simulink model "modelBCPWM"  (R2024a)
settings: Solver=ode23tb  StartTime=0.0  StopTime=0.05  MaxStep=sover_max_step  RelTol=1e-5
values from neighbouring files (symbols this model uses):
  BLDC_120_180 = 1    [initBCPWM.m]
  duty_cycle = 0.6    [initBCPWM.m]
  f_fundamental = 265    [initBCPWM.m]    (also in initSVPWM.m = 100)
  f_pwm = 20000    [initBCPWM.m]    (also in initSVPWM.m)
  Ke = sqrt(2) * 3.35e-3 * 60 / 2 / pi / p    [initBCPWM.m]    (also in initSVPWM.m)
  load_angle = pi/6    (= 0.523598775598)    [initBCPWM.m]    (also in initSVPWM.m = load_angle_offset - voltage_angle)
  Ls = 3/2 * 1.2e-3    (= 0.0018)    [initBCPWM.m]    (also in initSVPWM.m)
  Rs = 3/2 * 0.8    (= 1.2)    [initBCPWM.m]    (also in initSVPWM.m)
  sover_max_step = 1e-6    (= 1e-06)    [initBCPWM.m]    (also in initSVPWM.m)
  Vdc = 24    [initBCPWM.m]    (also in initSVPWM.m)
libraries: simulink x16, spsSeriesRLCBranchLib x6, spsMosfetLib x6, spsVoltageMeasurementLib x5, spsNeutralLib x4, spsControlledVoltageSourceLib x3, spsGroundLib x3, spsCurrentMeasurementLib x1, spsDCVoltageSourceLib x1, sps_lib x1
settings Model: SimulationMode=accelerator  Creator=mandr  LastModifiedBy=danielmcguiness
settings SolverCC: ZeroCrossControl=EnableAll  AlgebraicLoopSolver=TrustRegion  SolverResetMethod=Robust
settings DebuggingCC: UnconnectedInputMsg=warning  UnconnectedOutputMsg=warning  UnconnectedLineMsg=warning
settings ModelReferenceCC: EnableRefExpFcnMdlSchedulingChecks=on
settings RTWCC: GPUComputeCapability=3.5

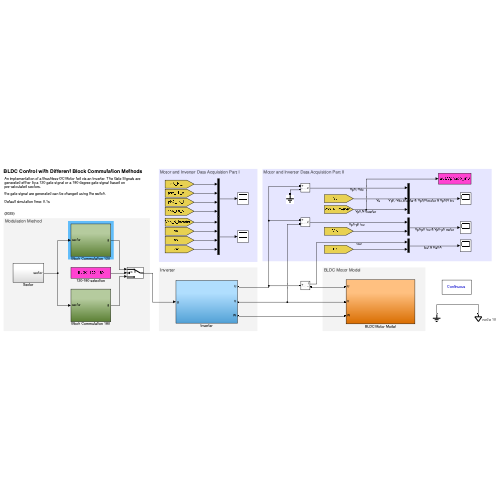
[thumbnail: Simulink's stored preview of the top-level diagram]
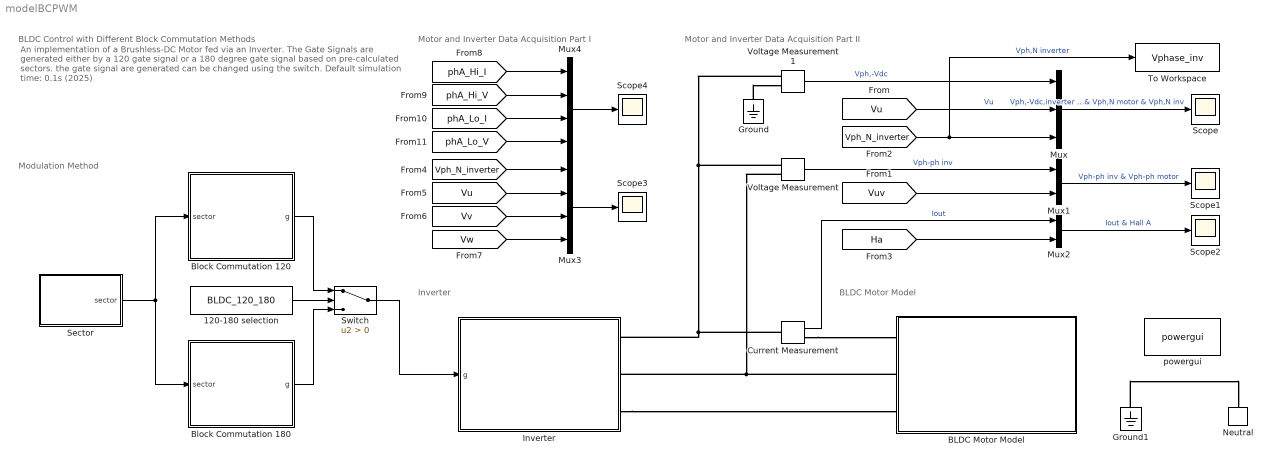
== system modelBCPWM ==
  note: An implementation of a Brushless-DC Motor fed via an Inverter. The Gate Signals are generated either by a 120 gate signal or a 180 degree gate signal based on
      | pre-calculated sectors.
      | the gate signal are generated can be changed using the switch.
      | Default simulation time: 0.1s
      |
      | (2025)
  note: BLDC Control with Different Block Commutation Methods
  note: BLDC Motor Model
  note: Motor and Inverter Data Acquisition Part II
  note: Motor and Inverter Data Acquisition Part I
  note: Inverter
  note: Modulation Method
  120-180 selection : Constant  Value=BLDC_120_180
  BLDC Motor Model : Subsystem
  Block Commutation 120 : Subsystem
  Block Commutation 180 : Subsystem
  Current Measurement : spsCurrentMeasurementLib/Current Measurement  PhasorSimulation=off  OutputType=Complex  PSBequivalent=0
  Ground : spsGroundLib/Ground  LConnTagsString=a
  Ground1 : spsGroundLib/Ground  LConnTagsString=a
  Inverter : Subsystem
  Mux : Mux  Inputs=3
  Mux1 : Mux  Inputs=2
  Mux2 : Mux  Inputs=2
  Mux3 : Mux
  Mux4 : Mux
  Neutral : spsNeutralLib/Neutral  LConnTagsString=a  NodeNumber=10
      settings: AttributesFormatString=node %<NodeNumber>  LibrarySourceBlock=sps_lib/Utilities/Neutral
  Scope{,1..4} (5 alike) : Scope
  Sector : Subsystem
  Switch : Switch  Criteria=u2 > Threshold  SaturateOnIntegerOverflow=off  InputSameDT=off
  To Workspace : ToWorkspace  VariableName=Vphase_inv  SaveFormat=Timeseries  SampleTime=sover_max_step
  Voltage Measurement : spsVoltageMeasurementLib/Voltage Measurement  PhasorSimulation=off  OutputType=Complex  PSBequivalent=0
  Voltage Measurement1 : spsVoltageMeasurementLib/Voltage Measurement  PhasorSimulation=off  OutputType=Complex  PSBequivalent=0
  powergui : sps_lib/powergui  Priority=1  SimulationMode=Continuous  SampleTime=50e-6  frequency=60  Iterations=50  frequencyindice=0  Pbase=100e6  ErrMax=1e-4  UnitsV=kV  UnitsW=MW  buscounter=0  FunctionMessages=off  echomessages=off  EnableUseOfTLC=off  CurrentSourceSwitches=off  DisableSnubberDevices=off  DisableRonSwitches=off  DisableVfSwitches=off  DisplayEquations=off  AutomaticDiscreteSolvers=off  SolverType=Tustin/Backward Euler (TBE)  Interpol=off  ExternalGateDelay=off  methode=off  Ts=100  x0status=blocks  SPID=on  SwTol=0  HookPort=off  NonlinearTolerance=1e-4  nMaxIteration=100  ContinueOnMaxIteration=off  RestoreLinks=warning  ResistiveCurrentMeasurement=off  Frange=[0:2:500]  Ylog=off  Xlog=on  ShowGrid=off  save=off  variable=ZData  structure=0  ZoomFFT=off  StartTime=0.0  cycles=1  DisplayStyle=1  fundamental=60  FreqAxis=off  MaxFrequency=1000  frequencyindicesteady=1  RmsSteady=1  display=off
  wires:
  Voltage Measurement1/1 -> Mux/1  "Vph,-Vdc"
  Voltage Measurement/1 -> Mux1/1  "Vph-ph inv"
  Current Measurement/1 -> Mux2/1  "Iout"
  Mux/1 -> Scope/1  "Vph,-Vdc,inverter & Vph,N motor & Vph,N inv"
  [Vu] -> Mux/2  "Vu"
  Mux1/1 -> Scope1/1  "Vph-ph inv & Vph-ph motor"
  [Vuv] -> Mux1/2
  [Vph_N_inverter] -> To Workspace/1, Mux/3  "Vph,N inverter"
  Mux2/1 -> Scope2/1  "Iout & Hall A"
  [Ha] -> Mux2/2
  Switch/1 -> Inverter/1(g)
  Block Commutation 180/1(g) -> Switch/3
  Block Commutation 120/1(g) -> Switch/1
  120-180 selection/1 -> Switch/2
  [Vph_N_inverter] -> Mux3/1
  Mux3/1 -> Scope3/1
  [Vu] -> Mux3/2
  [Vv] -> Mux3/3
  [Vw] -> Mux3/4
  Sector/1(sector) -> Block Commutation 180/1(sector), Block Commutation 120/1(sector)
  [phA_Hi_I] -> Mux4/1
  [phA_Hi_V] -> Mux4/2
  [phA_Lo_I] -> Mux4/3
  [phA_Lo_V] -> Mux4/4
  Mux4/1 -> Scope4/1
  connections:
  Voltage Measurement/LConn1 -- Current Measurement/LConn1 -- Inverter/RConn1 -- Voltage Measurement1/LConn1
  Voltage Measurement/LConn2 -- BLDC Motor Model/LConn2 -- Inverter/RConn2
  Ground/LConn1 -- Voltage Measurement1/LConn2
  Current Measurement/RConn1 -- BLDC Motor Model/LConn1
  Inverter/RConn3 -- BLDC Motor Model/LConn3
  Ground1/LConn1 -- Neutral/LConn1

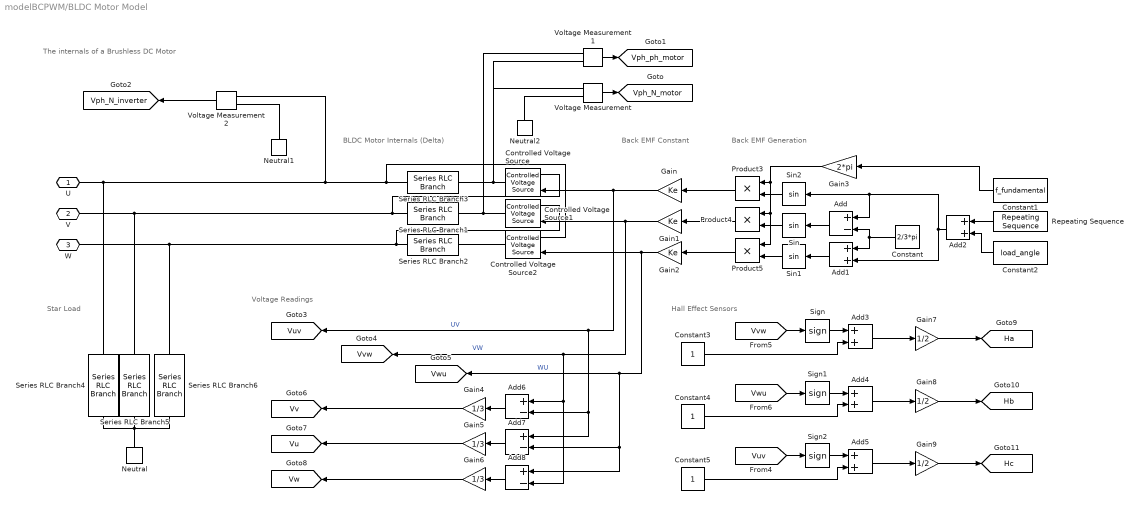
== system modelBCPWM/BLDC Motor Model ==
  note: The internals of a Brushless DC Motor
  note: Back EMF Generation
  note: Back EMF Constant
  note: Star Load
  note: Voltage Readings
  note: Hall Effect Sensors
  note: BLDC Motor Internals (Delta)
  Add{,6..8} (4 alike) : Sum  Inputs=+-
  Add{1..5} (5 alike) : Sum
  Constant : Constant  Value=2/3*pi
  Constant1 : Constant  Value=f_fundamental
  Constant2 : Constant  Value=load_angle
  Constant3 : Constant
  Constant4 : Constant
  Constant5 : Constant
  Controlled Voltage Source : spsControlledVoltageSourceLib/Controlled Voltage Source  Initialize=on  Source_Type=AC  Amplitude=0  Phase=0  Frequency=0  Measurements=None
  Controlled Voltage Source1 : spsControlledVoltageSourceLib/Controlled Voltage Source  Initialize=on  Source_Type=AC  Amplitude=0  Phase=0  Frequency=0  Measurements=None
  Controlled Voltage Source2 : spsControlledVoltageSourceLib/Controlled Voltage Source  Initialize=on  Source_Type=AC  Amplitude=0  Phase=0  Frequency=0  Measurements=None
  Gain : Gain  Gain=Ke
  Gain1 : Gain  Gain=Ke
  Gain2 : Gain  Gain=Ke
  Gain3 : Gain  Gain=2*pi
  Gain4 : Gain  Gain=1/3
  Gain5 : Gain  Gain=1/3
  Gain6 : Gain  Gain=1/3
  Gain7 : Gain  Gain=1/2
  Gain8 : Gain  Gain=1/2
  Gain9 : Gain  Gain=1/2
  Neutral : spsNeutralLib/Neutral  LConnTagsString=a  NodeNumber=10
      settings: AttributesFormatString=node %<NodeNumber>  LibrarySourceBlock=sps_lib/Utilities/Neutral
  Neutral1 : spsNeutralLib/Neutral  LConnTagsString=a  NodeNumber=10
      settings: AttributesFormatString=node %<NodeNumber>  LibrarySourceBlock=sps_lib/Utilities/Neutral
  Neutral2 : spsNeutralLib/Neutral  LConnTagsString=a  NodeNumber=10
      settings: AttributesFormatString=node %<NodeNumber>  LibrarySourceBlock=sps_lib/Utilities/Neutral
  Product3 : Product
  Product4 : Product
  Product5 : Product
  Repeating Sequence : simulink/Sources/Repeating Sequence  rep_seq_t=[0 1/f_fundamental]  rep_seq_y=[0 2*pi]
  Series RLC Branch1 : spsSeriesRLCBranchLib/Series RLC Branch  LConnTagsString=__new0  RConnTagsString=__new0  BranchType=RL  Resistance=Rs  Inductance=Ls  SetiL0=off  InitialCurrent=0  Capacitance=1e-6  Setx0=off  InitialVoltage=0  Measurements=None
  Series RLC Branch2 : spsSeriesRLCBranchLib/Series RLC Branch  LConnTagsString=__new0  RConnTagsString=__new0  BranchType=RL  Resistance=Rs  Inductance=Ls  SetiL0=off  InitialCurrent=0  Capacitance=1e-6  Setx0=off  InitialVoltage=0  Measurements=None
  Series RLC Branch3 : spsSeriesRLCBranchLib/Series RLC Branch  LConnTagsString=__new0  RConnTagsString=__new0  BranchType=RL  Resistance=Rs  Inductance=Ls  SetiL0=off  InitialCurrent=0  Capacitance=1e-6  Setx0=off  InitialVoltage=0  Measurements=None
  Series RLC Branch4 : spsSeriesRLCBranchLib/Series RLC Branch  LConnTagsString=__new0  RConnTagsString=__new0  BranchType=R  Resistance=1e3  Inductance=Ls  SetiL0=off  InitialCurrent=0  Capacitance=1e-6  Setx0=off  InitialVoltage=0  Measurements=None
  Series RLC Branch5 : spsSeriesRLCBranchLib/Series RLC Branch  LConnTagsString=__new0  RConnTagsString=__new0  BranchType=R  Resistance=1e3  Inductance=Ls  SetiL0=off  InitialCurrent=0  Capacitance=1e-6  Setx0=off  InitialVoltage=0  Measurements=None
  Series RLC Branch6 : spsSeriesRLCBranchLib/Series RLC Branch  LConnTagsString=__new0  RConnTagsString=__new0  BranchType=R  Resistance=1e3  Inductance=Ls  SetiL0=off  InitialCurrent=0  Capacitance=1e-6  Setx0=off  InitialVoltage=0  Measurements=None
  Sign : Signum
  Sign1 : Signum
  Sign2 : Signum
  Sin : Trigonometry
  Sin1 : Trigonometry
  Sin2 : Trigonometry
  Voltage Measurement : spsVoltageMeasurementLib/Voltage Measurement  PhasorSimulation=off  OutputType=Complex  PSBequivalent=0
  Voltage Measurement1 : spsVoltageMeasurementLib/Voltage Measurement  PhasorSimulation=off  OutputType=Complex  PSBequivalent=0
  Voltage Measurement2 : spsVoltageMeasurementLib/Voltage Measurement  PhasorSimulation=off  OutputType=Complex  PSBequivalent=0
  U : PMIOPort  Side=Left
  V : PMIOPort  Port=2  Side=Left
  W : PMIOPort  Port=3  Side=Left
  tag scope: Ha=global, Hb=global, Hc=global, Vph_N_inverter=global, Vph_N_motor=global, Vph_ph_motor=global, Vu=global, Vuv=global, Vv=global, Vvw=global, Vw=global, Vwu=global
  wires:
  Gain1/1 -> Add8/2, Add6/1, [Vvw], Controlled Voltage Source1/1  "VW"
  Product5/1 -> Gain2/1
  Gain/1 -> [Vuv], Add7/1, Add6/2, Controlled Voltage Source/1  "UV"
  Product3/1 -> Gain/1
  Constant/1 -> Add/2, Add1/1
  Product4/1 -> Gain1/1
  Gain2/1 -> Controlled Voltage Source2/1, Add8/1, Add7/2, [Vwu]  "WU"
  Add1/1 -> Sin1/1
  Add/1 -> Sin/1
  Sin2/1 -> Product3/2
  Sin/1 -> Product4/2
  Sin1/1 -> Product5/2
  Add2/1 -> Add/1, Sin2/1, Add1/2
  Constant1/1 -> Gain3/1
  Gain3/1 -> Product5/1, Product4/1, Product3/1
  Repeating Sequence/1 -> Add2/1
  Constant2/1 -> Add2/2
  Voltage Measurement/1 -> [Vph_N_motor]
  Voltage Measurement1/1 -> [Vph_ph_motor]
  Voltage Measurement2/1 -> [Vph_N_inverter]
  Add6/1 -> Gain4/1
  Gain4/1 -> [Vv]
  Add7/1 -> Gain5/1
  Gain5/1 -> [Vu]
  Add8/1 -> Gain6/1
  Gain6/1 -> [Vw]
  Add3/1 -> Gain7/1
  Sign/1 -> Add3/1
  Constant3/1 -> Add3/2
  [Vvw] -> Sign/1
  Gain7/1 -> [Ha]
  Gain8/1 -> [Hb]
  Constant4/1 -> Add4/2
  Sign1/1 -> Add4/1
  Add4/1 -> Gain8/1
  [Vwu] -> Sign1/1
  Add5/1 -> Gain9/1
  Sign2/1 -> Add5/1
  Constant5/1 -> Add5/2
  Gain9/1 -> [Hc]
  [Vuv] -> Sign2/1
  connections:
  U/RConn1 -- Voltage Measurement2/LConn1 -- Controlled Voltage Source2/LConn1 -- Series RLC Branch3/LConn1 -- Series RLC Branch4/LConn1
  V/RConn1 -- Controlled Voltage Source/LConn1 -- Series RLC Branch1/LConn1 -- Series RLC Branch5/LConn1
  W/RConn1 -- Series RLC Branch6/LConn1 -- Controlled Voltage Source1/LConn1 -- Series RLC Branch2/LConn1
  Series RLC Branch3/RConn1 -- Voltage Measurement1/LConn1 -- Voltage Measurement/LConn1 -- Controlled Voltage Source/RConn1
  Series RLC Branch1/RConn1 -- Voltage Measurement1/LConn2 -- Controlled Voltage Source1/RConn1
  Series RLC Branch2/RConn1 -- Controlled Voltage Source2/RConn1
  Series RLC Branch4/RConn1 -- Neutral/LConn1 -- Series RLC Branch5/RConn1 -- Series RLC Branch6/RConn1
  Voltage Measurement2/LConn2 -- Neutral1/LConn1
  Voltage Measurement/LConn2 -- Neutral2/LConn1

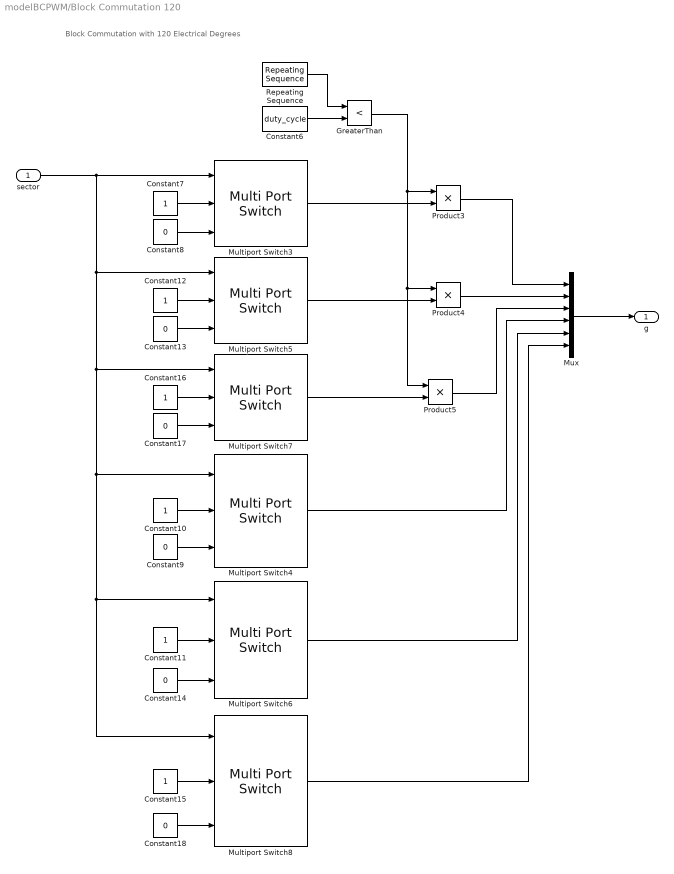
== system modelBCPWM/Block Commutation 120 ==
  note: Block Commutation with 120 Electrical Degrees
  sector : Inport
  Constant{7,10..12,15..16} (6 alike) : Constant
  Constant{8..9,13..14,17..18} (6 alike) : Constant  Value=0
  Constant6 : Constant  Value=duty_cycle
  GreaterThan : RelationalOperator  Operator=<  OutDataTypeStr=boolean  RndMeth=Simplest  InputSameDT=off
  Multiport Switch3 : MultiPortSwitch  DataPortOrder=Specify indices  Inputs=6  DataPortIndices={[1,2],[3,4,5,6]}  SaturateOnIntegerOverflow=off  InputSameDT=off
  Multiport Switch4 : MultiPortSwitch  DataPortOrder=Specify indices  Inputs=6  DataPortIndices={[4,5],[6,1,2,3]}  SaturateOnIntegerOverflow=off  InputSameDT=off
  Multiport Switch5 : MultiPortSwitch  DataPortOrder=Specify indices  Inputs=6  DataPortIndices={[3,4],[5,6,1,2]}  SaturateOnIntegerOverflow=off  InputSameDT=off
  Multiport Switch6 : MultiPortSwitch  DataPortOrder=Specify indices  Inputs=6  DataPortIndices={[6,1],[2,3,4,5]}  SaturateOnIntegerOverflow=off  InputSameDT=off
  Multiport Switch7 : MultiPortSwitch  DataPortOrder=Specify indices  Inputs=6  DataPortIndices={[5,6],[1,2,3,4]}  SaturateOnIntegerOverflow=off  InputSameDT=off
  Multiport Switch8 : MultiPortSwitch  DataPortOrder=Specify indices  Inputs=6  DataPortIndices={[2,3],[4,5,6,1]}  SaturateOnIntegerOverflow=off  InputSameDT=off
  Mux : Mux  Inputs=6
  Product3 : Product
  Product4 : Product
  Product5 : Product
  Repeating Sequence : simulink/Sources/Repeating Sequence  rep_seq_t=[0 1/f_pwm]  rep_seq_y=[0 1]
  g : Outport
  wires:
  Constant9/1 -> Multiport Switch4/3
  Multiport Switch5/1 -> Product4/2
  Multiport Switch3/1 -> Product3/2
  Multiport Switch8/1 -> Mux/6
  Multiport Switch6/1 -> Mux/5
  Product3/1 -> Mux/1
  Product4/1 -> Mux/2
  Multiport Switch7/1 -> Product5/2
  Multiport Switch4/1 -> Mux/4
  Mux/1 -> g/1
  Constant10/1 -> Multiport Switch4/2
  sector/1 -> Multiport Switch3/1, Multiport Switch8/1, Multiport Switch6/1, Multiport Switch4/1, Multiport Switch7/1, Multiport Switch5/1
  Constant15/1 -> Multiport Switch8/2
  Constant18/1 -> Multiport Switch8/3
  Constant17/1 -> Multiport Switch7/3
  Constant12/1 -> Multiport Switch5/2
  Repeating Sequence/1 -> GreaterThan/1
  Constant14/1 -> Multiport Switch6/3
  Constant11/1 -> Multiport Switch6/2
  Constant7/1 -> Multiport Switch3/2
  Constant8/1 -> Multiport Switch3/3
  Constant16/1 -> Multiport Switch7/2
  GreaterThan/1 -> Product3/1, Product5/1, Product4/1
  Product5/1 -> Mux/3
  Constant6/1 -> GreaterThan/2
  Constant13/1 -> Multiport Switch5/3

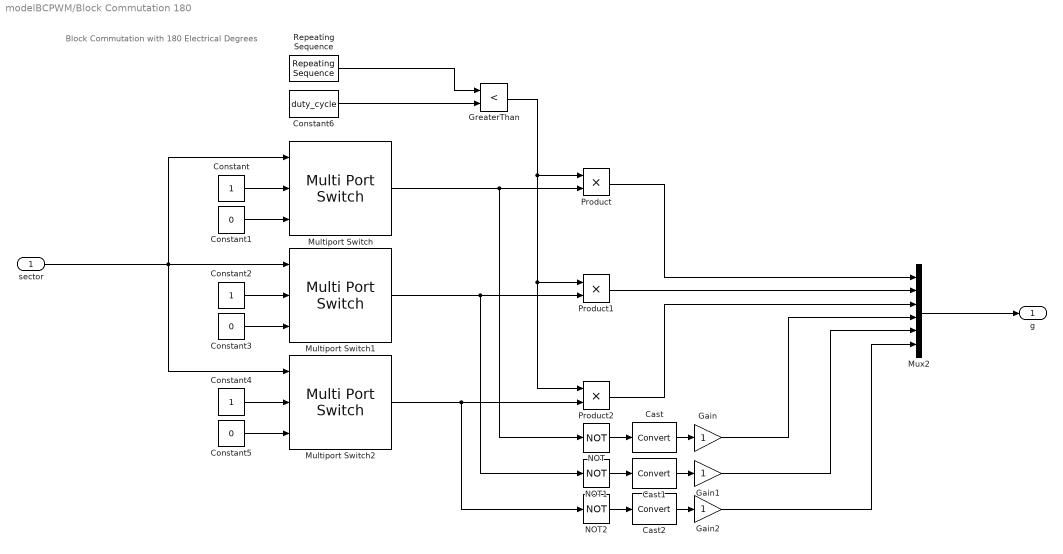
== system modelBCPWM/Block Commutation 180 ==
  note: Block Commutation with 180 Electrical Degrees
  sector : Inport
  Cast : DataTypeConversion  SaturateOnIntegerOverflow=off  RndMeth=Floor
  Cast1 : DataTypeConversion  SaturateOnIntegerOverflow=off  RndMeth=Floor
  Cast2 : DataTypeConversion  SaturateOnIntegerOverflow=off  RndMeth=Floor
  Constant : Constant
  Constant1 : Constant  Value=0
  Constant2 : Constant
  Constant3 : Constant  Value=0
  Constant4 : Constant
  Constant5 : Constant  Value=0
  Constant6 : Constant  Value=duty_cycle
  Gain : Gain
  Gain1 : Gain
  Gain2 : Gain
  GreaterThan : RelationalOperator  Operator=<  OutDataTypeStr=boolean  RndMeth=Simplest  InputSameDT=off
  Multiport Switch : MultiPortSwitch  DataPortOrder=Specify indices  Inputs=6  DataPortIndices={[1,2,3],[4,5,6]}  SaturateOnIntegerOverflow=off  InputSameDT=off
  Multiport Switch1 : MultiPortSwitch  DataPortOrder=Specify indices  Inputs=6  DataPortIndices={[3,4,5],[6,1,2]}  SaturateOnIntegerOverflow=off  InputSameDT=off
  Multiport Switch2 : MultiPortSwitch  DataPortOrder=Specify indices  Inputs=6  DataPortIndices={[5,6,1],[2,3,4]}  SaturateOnIntegerOverflow=off  InputSameDT=off
  Mux2 : Mux  Inputs=6
  NOT : Logic  Operator=NOT  AllPortsSameDT=off  OutDataTypeStr=boolean
  NOT1 : Logic  Operator=NOT  AllPortsSameDT=off  OutDataTypeStr=boolean
  NOT2 : Logic  Operator=NOT  AllPortsSameDT=off  OutDataTypeStr=boolean
  Product : Product
  Product1 : Product
  Product2 : Product
  Repeating Sequence : simulink/Sources/Repeating Sequence  rep_seq_t=[0 1/f_pwm]  rep_seq_y=[0 1]
  g : Outport
  wires:
  Constant4/1 -> Multiport Switch2/2
  GreaterThan/1 -> Product2/1, Product1/1, Product/1
  Constant/1 -> Multiport Switch/2
  Multiport Switch1/1 -> NOT1/1, Product1/2
  Multiport Switch/1 -> Product/2, NOT/1
  Constant1/1 -> Multiport Switch/3
  Repeating Sequence/1 -> GreaterThan/1
  Multiport Switch2/1 -> NOT2/1, Product2/2
  Product1/1 -> Mux2/2
  Constant6/1 -> GreaterThan/2
  Constant5/1 -> Multiport Switch2/3
  NOT/1 -> Cast/1
  Constant3/1 -> Multiport Switch1/3
  Constant2/1 -> Multiport Switch1/2
  Cast/1 -> Gain/1
  Product2/1 -> Mux2/3
  Product/1 -> Mux2/1
  sector/1 -> Multiport Switch/1, Multiport Switch2/1, Multiport Switch1/1
  Mux2/1 -> g/1
  Gain/1 -> Mux2/4
  Gain1/1 -> Mux2/5
  Gain2/1 -> Mux2/6
  Cast1/1 -> Gain1/1
  NOT1/1 -> Cast1/1
  NOT2/1 -> Cast2/1
  Cast2/1 -> Gain2/1

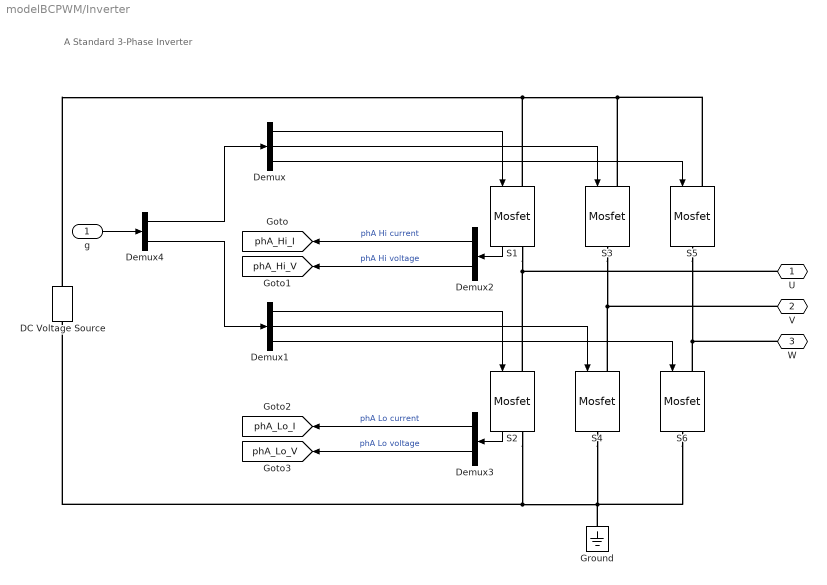
== system modelBCPWM/Inverter ==
  note: A Standard 3-Phase Inverter
  g : Inport
  DC Voltage Source : spsDCVoltageSourceLib/DC Voltage Source  Amplitude=Vdc  Measurements=None
  Demux : Demux  Outputs=3
  Demux1 : Demux  Outputs=3
  Demux2 : Demux  Outputs=2
  Demux3 : Demux  Outputs=2
  Demux4 : Demux  Outputs=2
  Ground : spsGroundLib/Ground  LConnTagsString=a
  S1 : spsMosfetLib/Mosfet  Ron=Ron  Lon=0  Rd=Rd  Vfd=Vf  IC=0  Rs=1e5  Cs=inf  Measurements=on
  S2 : spsMosfetLib/Mosfet  Ron=Ron  Lon=0  Rd=Rd  Vfd=Vf  IC=0  Rs=1e5  Cs=inf  Measurements=on
  S{3..6} (4 alike) : spsMosfetLib/Mosfet  Ron=Ron  Lon=0  Rd=Rd  Vfd=Vf  IC=0  Rs=1e5  Cs=inf  Measurements=off
  U : PMIOPort  Side=Right
  V : PMIOPort  Port=2  Side=Right
  W : PMIOPort  Port=3  Side=Right
  tag scope: phA_Hi_I=global, phA_Hi_V=global, phA_Lo_I=global, phA_Lo_V=global
  wires:
  Demux/3 -> S5/1
  Demux/1 -> S1/1
  Demux/2 -> S3/1
  Demux1/2 -> S4/1
  Demux1/1 -> S2/1
  Demux1/3 -> S6/1
  Demux3/1 -> [phA_Lo_I]  "phA Lo current"
  Demux3/2 -> [phA_Lo_V]  "phA Lo voltage"
  S2/1 -> Demux3/1
  S1/1 -> Demux2/1
  Demux2/1 -> [phA_Hi_I]  "phA Hi current"
  Demux2/2 -> [phA_Hi_V]  "phA Hi voltage"
  Demux4/1 -> Demux/1
  Demux4/2 -> Demux1/1
  g/1 -> Demux4/1
  connections:
  DC Voltage Source/RConn1 -- S5/LConn1 -- S3/LConn1 -- S1/LConn1
  S1/RConn1 -- S2/LConn1 -- U/RConn1
  DC Voltage Source/LConn1 -- S2/RConn1 -- S6/RConn1 -- Ground/LConn1 -- S4/RConn1
  W/RConn1 -- S6/LConn1 -- S5/RConn1
  V/RConn1 -- S3/RConn1 -- S4/LConn1

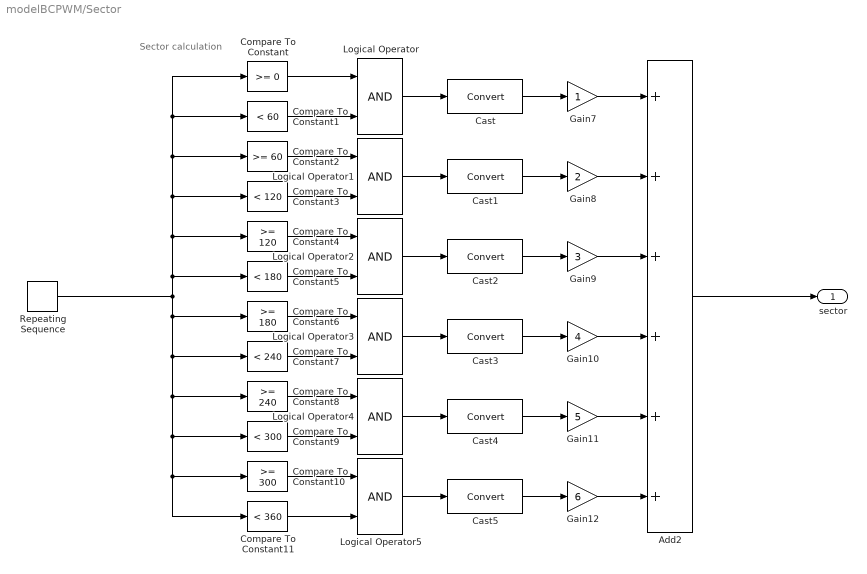
== system modelBCPWM/Sector ==
  note: Sector calculation
  Add2 : Sum  Inputs=6
  Cast{,1..5} (6 alike) : DataTypeConversion  SaturateOnIntegerOverflow=off  RndMeth=Floor
  Compare To Constant : simulink/Logic and Bit Operations/Compare To Constant  relop=>=  const=0  OutDataTypeStr=boolean
  Compare To Constant1 : simulink/Logic and Bit Operations/Compare To Constant  relop=<  const=60  OutDataTypeStr=boolean
  Compare To Constant10 : simulink/Logic and Bit Operations/Compare To Constant  relop=>=  const=300  OutDataTypeStr=boolean
  Compare To Constant11 : simulink/Logic and Bit Operations/Compare To Constant  relop=<  const=360  OutDataTypeStr=boolean
  Compare To Constant2 : simulink/Logic and Bit Operations/Compare To Constant  relop=>=  const=60  OutDataTypeStr=boolean
  Compare To Constant3 : simulink/Logic and Bit Operations/Compare To Constant  relop=<  const=120  OutDataTypeStr=boolean
  Compare To Constant4 : simulink/Logic and Bit Operations/Compare To Constant  relop=>=  const=120  OutDataTypeStr=boolean
  Compare To Constant5 : simulink/Logic and Bit Operations/Compare To Constant  relop=<  const=180  OutDataTypeStr=boolean
  Compare To Constant6 : simulink/Logic and Bit Operations/Compare To Constant  relop=>=  const=180  OutDataTypeStr=boolean
  Compare To Constant7 : simulink/Logic and Bit Operations/Compare To Constant  relop=<  const=240  OutDataTypeStr=boolean
  Compare To Constant8 : simulink/Logic and Bit Operations/Compare To Constant  relop=>=  const=240  OutDataTypeStr=boolean
  Compare To Constant9 : simulink/Logic and Bit Operations/Compare To Constant  relop=<  const=300  OutDataTypeStr=boolean
  Gain10 : Gain  Gain=4
  Gain11 : Gain  Gain=5
  Gain12 : Gain  Gain=6
  Gain7 : Gain
  Gain8 : Gain  Gain=2
  Gain9 : Gain  Gain=3
  Logical Operator{,1..5} (6 alike) : Logic  AllPortsSameDT=off  OutDataTypeStr=boolean
  Repeating Sequence : simulink/Sources/Repeating Sequence  rep_seq_t=[0 1/f_fundamental]  rep_seq_y=[0 360]
  sector : Outport
  wires:
  Cast/1 -> Gain7/1
  Compare To Constant11/1 -> Logical Operator5/2
  Logical Operator1/1 -> Cast1/1
  Compare To Constant4/1 -> Logical Operator2/1
  Cast4/1 -> Gain11/1
  Cast5/1 -> Gain12/1
  Logical Operator/1 -> Cast/1
  Repeating Sequence/1 -> Compare To Constant6/1, Compare To Constant8/1, Compare To Constant10/1, Compare To Constant11/1, Compare To Constant9/1, Compare To Constant7/1, Compare To Constant5/1, Compare To Constant4/1, Compare To Constant3/1, Compare To Constant/1, Compare To Constant1/1, Compare To Constant2/1
  Logical Operator3/1 -> Cast3/1
  Logical Operator4/1 -> Cast4/1
  Compare To Constant/1 -> Logical Operator/1
  Compare To Constant1/1 -> Logical Operator/2
  Gain8/1 -> Add2/2
  Logical Operator5/1 -> Cast5/1
  Compare To Constant6/1 -> Logical Operator3/1
  Gain9/1 -> Add2/3
  Cast2/1 -> Gain9/1
  Gain7/1 -> Add2/1
  Compare To Constant9/1 -> Logical Operator4/2
  Gain12/1 -> Add2/6
  Gain11/1 -> Add2/5
  Compare To Constant10/1 -> Logical Operator5/1
  Cast3/1 -> Gain10/1
  Compare To Constant3/1 -> Logical Operator1/2
  Compare To Constant2/1 -> Logical Operator1/1
  Gain10/1 -> Add2/4
  Compare To Constant5/1 -> Logical Operator2/2
  Compare To Constant7/1 -> Logical Operator3/2
  Compare To Constant8/1 -> Logical Operator4/1
  Logical Operator2/1 -> Cast2/1
  Cast1/1 -> Gain8/1
  Add2/1 -> sector/1
